simulink model "Challenge_errorspace"  (R2021a)
settings: Solver=ode45  StartTime=0.0  StopTime=1  RelTol=1e-3
undefined symbols (not defined in the file): challerr, degs2rpm, rpm2rads, sens
settings Model: Creator=gioel  LastModifiedBy=gioel

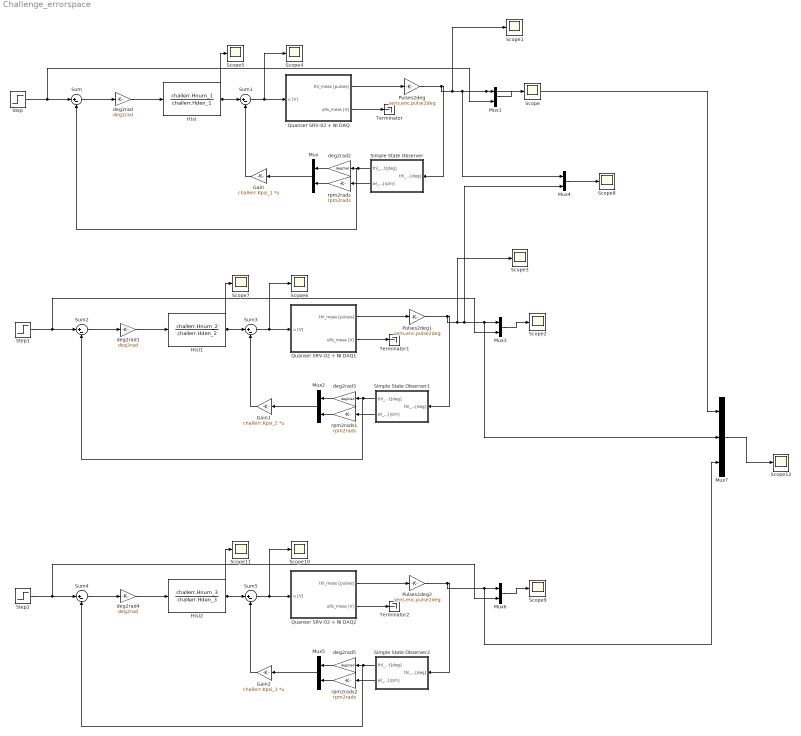
== system Challenge_errorspace ==
  Gain : Gain  Gain=challerr.Kpsi_1  Multiplication=Matrix(K*u)
  Gain1 : Gain  Gain=challerr.Kpsi_2  Multiplication=Matrix(K*u)
  Gain2 : Gain  Gain=challerr.Kpsi_3  Multiplication=Matrix(K*u)
  H(s) : TransferFcn  Numerator=challerr.Hnum_1  Denominator=challerr.Hden_1
  H(s)1 : TransferFcn  Numerator=challerr.Hnum_2  Denominator=challerr.Hden_2
  H(s)2 : TransferFcn  Numerator=challerr.Hnum_3  Denominator=challerr.Hden_3
  Mux{,1..6} (7 alike) : Mux  Inputs=2
  Mux7 : Mux  Inputs=3
  Pulses2deg : Gain  Gain=sens.enc.pulse2deg
  Pulses2deg1 : Gain  Gain=sens.enc.pulse2deg
  Pulses2deg2 : Gain  Gain=sens.enc.pulse2deg
  Quanser SRV-02 + NI DAQ : Subsystem  mask(Quanser SRV-02 (with inertial load) + NI DAQ){Ts=0.001, fricType=Karnopp}
      mask prompts: Ts "NI DAQ Sample Time:"; fricType "Friction model"
      mask help: Quanser SRV-02 (with inertial load) + NI DAQ model.
      mask init:
      | %%  Sensors data
      | 
      | %   shunt resistor
      | sens.curr.Rs = 0.5;                         %   resistance [Ohm]   
      | sens.curr.uRs_std = 0.01;                   %   voltage noise standard dev [V]                           
      | sens.curr.uRs_var = sens.curr.uRs_std^2;	%   voltage noise variance [V^2]
      | 
      | %   Hewlett-Packard HEDS-5540#A06 optical encoder
      | sens.enc.ppr = 500*4;                       %   pulses per rotation
      | sens.enc.pulse2deg = 360/sens.enc.ppr;      %   [pulses] -> [deg]
      | sens.enc.pulse2rad = 2*pi/sens.enc.ppr;     %   [pulses] -> [rad]
      | sens.enc.deg2pulse = sens.enc.ppr/360;      %   [deg] -> [pulses]
      | sens.enc.rad2pulse = sens.enc.ppr/2/pi;     %   [rad] -> [pulses]
      | 
      | 
      | %%  Data acquisition board (daq) data
      | 
      | %   NI PCI-6221 DAC data
      | daq.dac.bits = 16;                                  %   resolution (bits)
      | daq.dac.fs   = 10;                                  %   full scale 
      | daq.dac.q    = 2*daq.dac.fs/(2^daq.dac.bits-1);     %	quantization
      | 
      | %   NI PCI-6221 ADC data
      | daq.adc.bits = 16;                                  %   resolution (bits)
      | daq.adc.fs   = 10;                                  %   full scale (as set in SLDRT Analog Input block)
      | daq.adc.q    = 2*daq.adc.fs/(2^daq.adc.bits-1);     %   quantization
      mask Help:
      | Riccardo Antonello (antonello@dei.unipd.it)
      | 
      | April 24, 2020
      | 
      | Dept. of Information Engineering, University of Padova
      mask TypeOptions fricType: Coulomb + viscous | Karnopp
  Quanser SRV-02 + NI DAQ1 : Subsystem  mask(Quanser SRV-02 (with inertial load) + NI DAQ){Ts=0.001, fricType=Karnopp}
      mask prompts: Ts "NI DAQ Sample Time:"; fricType "Friction model"
      mask help: Quanser SRV-02 (with inertial load) + NI DAQ model.
      mask init: same as Challenge_errorspace/Quanser SRV-02 + NI DAQ
      mask Help:
      | Riccardo Antonello (antonello@dei.unipd.it)
      | 
      | April 24, 2020
      | 
      | Dept. of Information Engineering, University of Padova
      mask TypeOptions fricType: Coulomb + viscous | Karnopp
  Quanser SRV-02 + NI DAQ2 : Subsystem  mask(Quanser SRV-02 (with inertial load) + NI DAQ){Ts=0.001, fricType=Karnopp}
      mask prompts: Ts "NI DAQ Sample Time:"; fricType "Friction model"
      mask help: Quanser SRV-02 (with inertial load) + NI DAQ model.
      mask init: same as Challenge_errorspace/Quanser SRV-02 + NI DAQ
      mask Help:
      | Riccardo Antonello (antonello@dei.unipd.it)
      | 
      | April 24, 2020
      | 
      | Dept. of Information Engineering, University of Padova
      mask TypeOptions fricType: Coulomb + viscous | Karnopp
  Scope{,1..12} (13 alike) : Scope
  Simple State Observer : Subsystem
  Simple State Observer1 : Subsystem
  Simple State Observer2 : Subsystem
  Step : Step  Time=0  After=70  SampleTime=0
  Step1 : Step  Time=0  After=70  SampleTime=0
  Step2 : Step  Time=0  After=70  SampleTime=0
  Sum{,1..5} (6 alike) : Sum  Inputs=|+-
  Terminator : Terminator
  Terminator1 : Terminator
  Terminator2 : Terminator
  deg2rad{,1..5} (6 alike) : Gain  Gain=deg2rad
  rpm2rads : Gain  Gain=rpm2rads
  rpm2rads1 : Gain  Gain=rpm2rads
  rpm2rads2 : Gain  Gain=rpm2rads
  wires:
  Quanser SRV-02 + NI DAQ/2(uRs_meas [V]) -> Terminator/1
  Step/1 -> Mux1/2, Sum/1
  Quanser SRV-02 + NI DAQ/1(thl_meas [pulses]) -> Pulses2deg/1
  Mux/1 -> Gain/1
  Sum1/1 -> Scope4/1, Quanser SRV-02 + NI DAQ/1(u [V])
  H(s)/1 -> Scope5/1, Sum1/1
  Gain/1 -> Sum1/2
  Pulses2deg/1 -> Scope1/1, Mux4/1, Mux7/1, Mux1/1, Simple State Observer/1(thl_meas[deg])
  deg2rad/1 -> H(s)/1
  Sum/1 -> deg2rad/1
  deg2rad2/1 -> Mux/1
  Simple State Observer/1(thl_est[deg]) -> Sum/2, deg2rad2/1
  rpm2rads/1 -> Mux/2
  Simple State Observer/2(wl_est[rpm]) -> rpm2rads/1
  Mux1/1 -> Scope/1
  H(s)1/1 -> Scope7/1, Sum3/1
  Step1/1 -> Mux3/2, Sum2/1
  Mux2/1 -> Gain1/1
  Sum3/1 -> Scope6/1, Quanser SRV-02 + NI DAQ1/1(u [V])
  Quanser SRV-02 + NI DAQ1/1(thl_meas [pulses]) -> Pulses2deg1/1
  Quanser SRV-02 + NI DAQ1/2(uRs_meas [V]) -> Terminator1/1
  Gain1/1 -> Sum3/2
  Pulses2deg1/1 -> Scope3/1, Mux4/2, Mux7/2, Mux3/1, Simple State Observer1/1(thl_meas[deg])
  deg2rad3/1 -> Mux2/1
  rpm2rads1/1 -> Mux2/2
  Sum2/1 -> deg2rad1/1
  Mux3/1 -> Scope2/1
  Simple State Observer1/2(wl_est[rpm]) -> rpm2rads1/1
  Simple State Observer1/1(thl_est[deg]) -> Sum2/2, deg2rad3/1
  deg2rad1/1 -> H(s)1/1
  Mux4/1 -> Scope8/1
  deg2rad5/1 -> Mux5/1
  Simple State Observer2/2(wl_est[rpm]) -> rpm2rads2/1
  Sum4/1 -> deg2rad4/1
  Mux5/1 -> Gain2/1
  Step2/1 -> Mux6/2, Sum4/1
  Sum5/1 -> Scope10/1, Quanser SRV-02 + NI DAQ2/1(u [V])
  H(s)2/1 -> Scope11/1, Sum5/1
  rpm2rads2/1 -> Mux5/2
  Pulses2deg2/1 -> Mux7/3, Mux6/1, Simple State Observer2/1(thl_meas[deg])
  Gain2/1 -> Sum5/2
  Quanser SRV-02 + NI DAQ2/2(uRs_meas [V]) -> Terminator2/1
  Mux6/1 -> Scope9/1
  Quanser SRV-02 + NI DAQ2/1(thl_meas [pulses]) -> Pulses2deg2/1
  Simple State Observer2/1(thl_est[deg]) -> Sum4/2, deg2rad5/1
  deg2rad4/1 -> H(s)2/1
  Mux7/1 -> Scope12/1

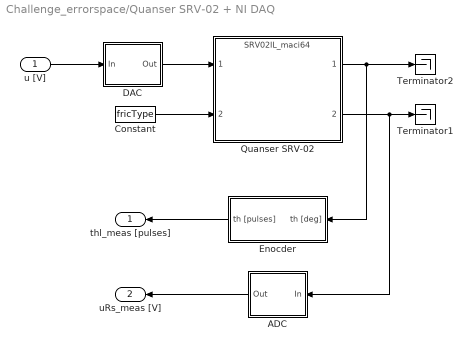
== system Challenge_errorspace/Quanser SRV-02 + NI DAQ ==
  u [V] : Inport
  ADC : Subsystem
  Constant : Constant  Value=fricType
  DAC : Subsystem
  Enocder : Subsystem
  Quanser SRV-02 : ModelReference  ModelNameDialog=SRV02IL_maci64.slxp  ModelReferenceVersion=1.44  CopyOfModelProtected=on
  Terminator1 : Terminator
  Terminator2 : Terminator
  thl_meas [pulses] : Outport
  uRs_meas [V] : Outport  Port=2
  wires:
  Enocder/1(th [pulses]) -> thl_meas [pulses]/1
  ADC/1(Out) -> uRs_meas [V]/1
  DAC/1(Out) -> Quanser SRV-02/1
  Quanser SRV-02/2 -> ADC/1(In), Terminator1/1
  u [V]/1 -> DAC/1(In)
  Quanser SRV-02/1 -> Enocder/1(th [deg]), Terminator2/1
  Constant/1 -> Quanser SRV-02/2

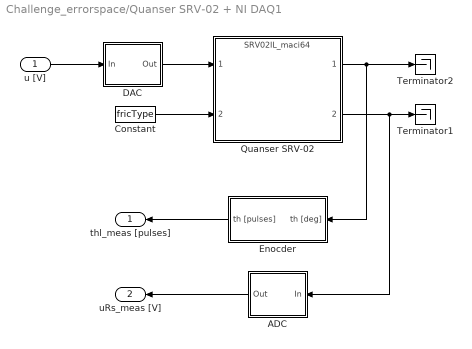
== system Challenge_errorspace/Quanser SRV-02 + NI DAQ1 ==
  u [V] : Inport
  ADC : Subsystem
  Constant : Constant  Value=fricType
  DAC : Subsystem
  Enocder : Subsystem
  Quanser SRV-02 : ModelReference  ModelNameDialog=SRV02IL_maci64.slxp  ModelReferenceVersion=1.44  CopyOfModelProtected=on
  Terminator1 : Terminator
  Terminator2 : Terminator
  thl_meas [pulses] : Outport
  uRs_meas [V] : Outport  Port=2
  wires:
  Enocder/1(th [pulses]) -> thl_meas [pulses]/1
  ADC/1(Out) -> uRs_meas [V]/1
  DAC/1(Out) -> Quanser SRV-02/1
  Quanser SRV-02/2 -> ADC/1(In), Terminator1/1
  u [V]/1 -> DAC/1(In)
  Quanser SRV-02/1 -> Enocder/1(th [deg]), Terminator2/1
  Constant/1 -> Quanser SRV-02/2

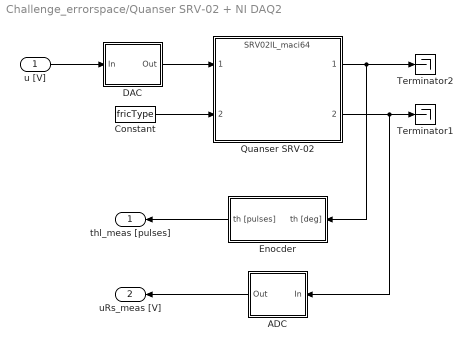
== system Challenge_errorspace/Quanser SRV-02 + NI DAQ2 ==
  u [V] : Inport
  ADC : Subsystem
  Constant : Constant  Value=fricType
  DAC : Subsystem
  Enocder : Subsystem
  Quanser SRV-02 : ModelReference  ModelNameDialog=SRV02IL_maci64.slxp  ModelReferenceVersion=1.44  CopyOfModelProtected=on
  Terminator1 : Terminator
  Terminator2 : Terminator
  thl_meas [pulses] : Outport
  uRs_meas [V] : Outport  Port=2
  wires:
  Enocder/1(th [pulses]) -> thl_meas [pulses]/1
  ADC/1(Out) -> uRs_meas [V]/1
  DAC/1(Out) -> Quanser SRV-02/1
  Quanser SRV-02/2 -> ADC/1(In), Terminator1/1
  u [V]/1 -> DAC/1(In)
  Quanser SRV-02/1 -> Enocder/1(th [deg]), Terminator2/1
  Constant/1 -> Quanser SRV-02/2

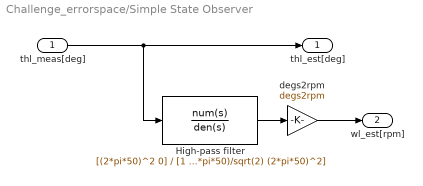
== system Challenge_errorspace/Simple State Observer ==
  thl_meas[deg] : Inport
  High-pass filter : TransferFcn  Numerator=[(2*pi*50)^2 0]  Denominator=[1 (2*2*pi*50)/sqrt(2) (2*pi*50)^2]
  degs2rpm : Gain  Gain=degs2rpm
  thl_est[deg] : Outport
  wl_est[rpm] : Outport  Port=2
  wires:
  High-pass filter/1 -> degs2rpm/1
  degs2rpm/1 -> wl_est[rpm]/1
  thl_meas[deg]/1 -> thl_est[deg]/1, High-pass filter/1

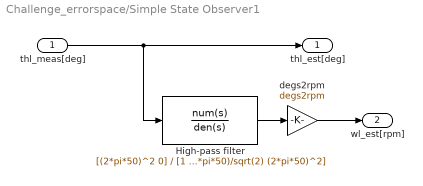
== system Challenge_errorspace/Simple State Observer1 ==
  thl_meas[deg] : Inport
  High-pass filter : TransferFcn  Numerator=[(2*pi*50)^2 0]  Denominator=[1 (2*2*pi*50)/sqrt(2) (2*pi*50)^2]
  degs2rpm : Gain  Gain=degs2rpm
  thl_est[deg] : Outport
  wl_est[rpm] : Outport  Port=2
  wires:
  High-pass filter/1 -> degs2rpm/1
  degs2rpm/1 -> wl_est[rpm]/1
  thl_meas[deg]/1 -> thl_est[deg]/1, High-pass filter/1

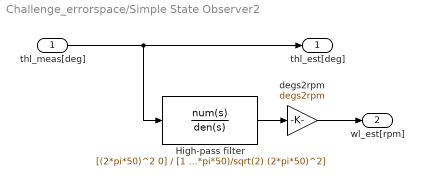
== system Challenge_errorspace/Simple State Observer2 ==
  thl_meas[deg] : Inport
  High-pass filter : TransferFcn  Numerator=[(2*pi*50)^2 0]  Denominator=[1 (2*2*pi*50)/sqrt(2) (2*pi*50)^2]
  degs2rpm : Gain  Gain=degs2rpm
  thl_est[deg] : Outport
  wl_est[rpm] : Outport  Port=2
  wires:
  High-pass filter/1 -> degs2rpm/1
  degs2rpm/1 -> wl_est[rpm]/1
  thl_meas[deg]/1 -> thl_est[deg]/1, High-pass filter/1

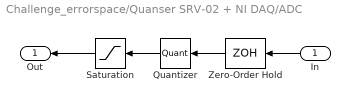
== system Challenge_errorspace/Quanser SRV-02 + NI DAQ/ADC ==
  In : Inport
  Quantizer : Quantizer  QuantizationInterval=daq.adc.q
  Saturation : Saturate  UpperLimit=daq.adc.fs  LowerLimit=-daq.adc.fs
  Zero-Order Hold : ZeroOrderHold  SampleTime=Ts
  Out : Outport
  wires:
  Saturation/1 -> Out/1
  In/1 -> Zero-Order Hold/1
  Quantizer/1 -> Saturation/1
  Zero-Order Hold/1 -> Quantizer/1

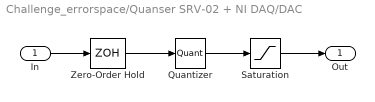
== system Challenge_errorspace/Quanser SRV-02 + NI DAQ/DAC ==
  In : Inport
  Quantizer : Quantizer  QuantizationInterval=daq.dac.q
  Saturation : Saturate  UpperLimit=daq.dac.fs  LowerLimit=-daq.dac.fs
  Zero-Order Hold : ZeroOrderHold  SampleTime=Ts
  Out : Outport
  wires:
  Quantizer/1 -> Saturation/1
  In/1 -> Zero-Order Hold/1
  Zero-Order Hold/1 -> Quantizer/1
  Saturation/1 -> Out/1

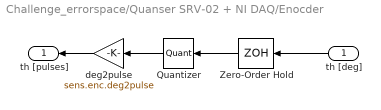
== system Challenge_errorspace/Quanser SRV-02 + NI DAQ/Enocder ==
  th [deg] : Inport
  Quantizer : Quantizer  QuantizationInterval=sens.enc.pulse2deg
  Zero-Order Hold : ZeroOrderHold  SampleTime=Ts
  deg2pulse : Gain  Gain=sens.enc.deg2pulse
  th [pulses] : Outport
  wires:
  Quantizer/1 -> deg2pulse/1
  th [deg]/1 -> Zero-Order Hold/1
  Zero-Order Hold/1 -> Quantizer/1
  deg2pulse/1 -> th [pulses]/1

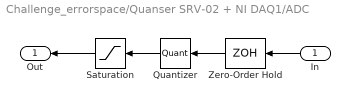
== system Challenge_errorspace/Quanser SRV-02 + NI DAQ1/ADC ==
  In : Inport
  Quantizer : Quantizer  QuantizationInterval=daq.adc.q
  Saturation : Saturate  UpperLimit=daq.adc.fs  LowerLimit=-daq.adc.fs
  Zero-Order Hold : ZeroOrderHold  SampleTime=Ts
  Out : Outport
  wires:
  Saturation/1 -> Out/1
  In/1 -> Zero-Order Hold/1
  Quantizer/1 -> Saturation/1
  Zero-Order Hold/1 -> Quantizer/1

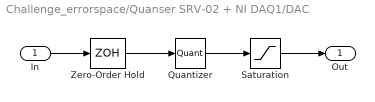
== system Challenge_errorspace/Quanser SRV-02 + NI DAQ1/DAC ==
  In : Inport
  Quantizer : Quantizer  QuantizationInterval=daq.dac.q
  Saturation : Saturate  UpperLimit=daq.dac.fs  LowerLimit=-daq.dac.fs
  Zero-Order Hold : ZeroOrderHold  SampleTime=Ts
  Out : Outport
  wires:
  Quantizer/1 -> Saturation/1
  In/1 -> Zero-Order Hold/1
  Zero-Order Hold/1 -> Quantizer/1
  Saturation/1 -> Out/1

== system Challenge_errorspace/Quanser SRV-02 + NI DAQ1/Enocder ==
  th [deg] : Inport
  Quantizer : Quantizer  QuantizationInterval=sens.enc.pulse2deg
  Zero-Order Hold : ZeroOrderHold  SampleTime=Ts
  deg2pulse : Gain  Gain=sens.enc.deg2pulse
  th [pulses] : Outport
  wires:
  Quantizer/1 -> deg2pulse/1
  th [deg]/1 -> Zero-Order Hold/1
  Zero-Order Hold/1 -> Quantizer/1
  deg2pulse/1 -> th [pulses]/1

== system Challenge_errorspace/Quanser SRV-02 + NI DAQ2/ADC ==
  In : Inport
  Quantizer : Quantizer  QuantizationInterval=daq.adc.q
  Saturation : Saturate  UpperLimit=daq.adc.fs  LowerLimit=-daq.adc.fs
  Zero-Order Hold : ZeroOrderHold  SampleTime=Ts
  Out : Outport
  wires:
  Saturation/1 -> Out/1
  In/1 -> Zero-Order Hold/1
  Quantizer/1 -> Saturation/1
  Zero-Order Hold/1 -> Quantizer/1

== system Challenge_errorspace/Quanser SRV-02 + NI DAQ2/DAC ==
  In : Inport
  Quantizer : Quantizer  QuantizationInterval=daq.dac.q
  Saturation : Saturate  UpperLimit=daq.dac.fs  LowerLimit=-daq.dac.fs
  Zero-Order Hold : ZeroOrderHold  SampleTime=Ts
  Out : Outport
  wires:
  Quantizer/1 -> Saturation/1
  In/1 -> Zero-Order Hold/1
  Zero-Order Hold/1 -> Quantizer/1
  Saturation/1 -> Out/1

== system Challenge_errorspace/Quanser SRV-02 + NI DAQ2/Enocder ==
  th [deg] : Inport
  Quantizer : Quantizer  QuantizationInterval=sens.enc.pulse2deg
  Zero-Order Hold : ZeroOrderHold  SampleTime=Ts
  deg2pulse : Gain  Gain=sens.enc.deg2pulse
  th [pulses] : Outport
  wires:
  Quantizer/1 -> deg2pulse/1
  th [deg]/1 -> Zero-Order Hold/1
  Zero-Order Hold/1 -> Quantizer/1
  deg2pulse/1 -> th [pulses]/1
